simulink model "model"  (Simulink 8.7)
settings: Solver=ode45  StartTime=0.0  StopTime=3000.0  RelTol=1e-3
libraries: commnoisgen2 x2
settings Model: Creator=a  LastModifiedBy=dous12
settings DebuggingCC: UnderspecifiedInitializationDetection=Simplified  MergeDetectMultiDrivingBlocksExec=error  SolverPrmCheckMsg=warning  AllowSymbolicDim=off
settings ConfigComp: CovSFcnEnable=off

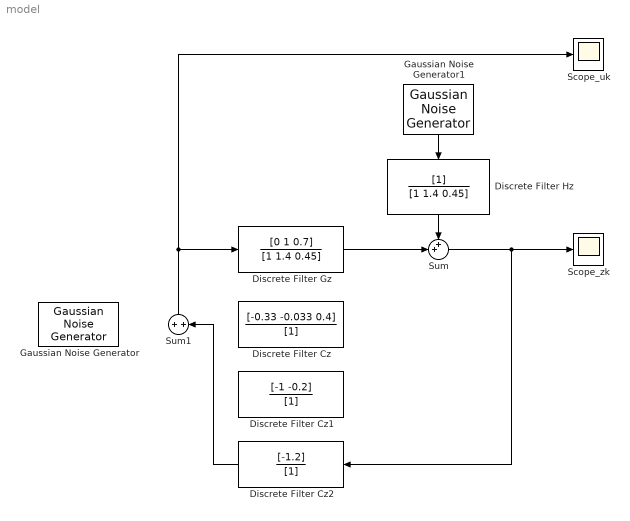
== system model ==
  Discrete Filter Cz : DiscreteFilter  Numerator=[-0.33 -0.033 0.4]  Denominator=[1]  SampleTime=1
  Discrete Filter Cz1 : DiscreteFilter  Numerator=[-1 -0.2]  Denominator=[1]
  Discrete Filter Cz2 : DiscreteFilter  Numerator=[-1.2]  Denominator=[1]
  Discrete Filter Gz : DiscreteFilter  Numerator=[0 1 0.7]  Denominator=[1 1.4 0.45]  SampleTime=1
  Discrete Filter Hz : DiscreteFilter  Denominator=[1 1.4 0.45]  SampleTime=1
  Gaussian Noise Generator : commnoisgen2/Gaussian Noise Generator  m=0  d=1  s=41  Ts=10  frameBased=off  sampPerFrame=1  orient=off  outDataType=double
  Gaussian Noise Generator1 : commnoisgen2/Gaussian Noise Generator  m=0  d=1  s=777  Ts=1  frameBased=off  sampPerFrame=1  orient=off  outDataType=double
  Scope_uk : Scope
  Scope_zk : Scope
  Sum : Sum  Inputs=++|
  Sum1 : Sum  Inputs=+|+
  wires:
  Gaussian Noise Generator1/1 -> Discrete Filter Hz/1
  Discrete Filter Gz/1 -> Sum/2
  Discrete Filter Hz/1 -> Sum/1
  Sum1/1 -> Scope_uk/1, Discrete Filter Gz/1
  Sum/1 -> Discrete Filter Cz2/1, Scope_zk/1
  Discrete Filter Cz2/1 -> Sum1/2
